simulink model "gm_uz_pmsm_model_9ph_vnl"  (R2021b)
settings: Solver=FixedStepAuto  StartTime=0.0  StopTime=0.8  RelTol=1e-3
PreLoadFcn:
  | uz_pmsm_model_9ph_init_parameter
undefined symbols (not defined in the file or in its folder): a, b, c, friction_coefficient, inertia, k_i_d, k_i_q, k_p_d, k_p_q, Kpd, L_d, L_o1, L_o2, L_q, L_x1, L_x2, L_y1, L_y2, L_zero, polepair, psi_pm, R_1, static_friction_torque, Tnd, ts
libraries: hdlmdlgenlib x191, hdlsllib x90, dspsigops x19, simulink x17, slpidlib x2, spsAlphaBetaZerotodq0Lib x1, pid_lib x1, spsdq0toAlphaBetaZeroLib x1
(part 5 of 7)

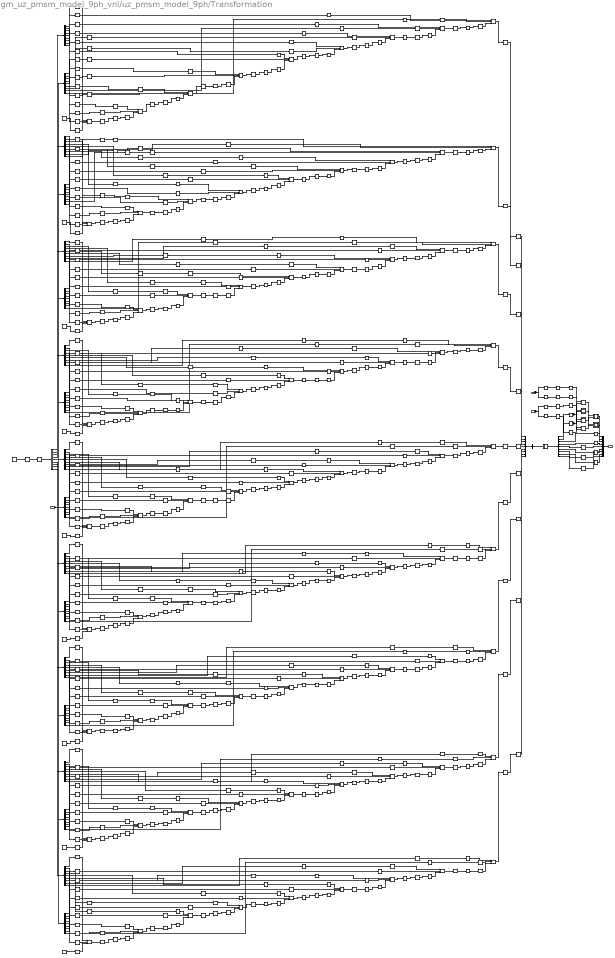
== system gm_uz_pmsm_model_9ph_vnl/uz_pmsm_model_9ph/Transformation ==
  in : Inport  OutDataTypeStr=fixdt(1, 25, 12)  PortDimensions=[9]  SampleTime=1e-08
  sin_theta_el : Inport  Port=2  OutDataTypeStr=single  SampleTime=1e-08
  cos_theta_el : Inport  Port=3  OutDataTypeStr=single  SampleTime=1e-08
  Add : Subsystem
      mask Display: disp('NFP\nadd');
  Add1 : Subsystem
      mask Display: disp('NFP\nadd');
  Constant1 : Constant  Value=[0.22222137451171875;0;0.22222137451171875;0;0.22222137451171875;0;0.22222137451171875;0;0.111110687255859375;-0.111110687255859375;0.1924495697021484375;0.22222137451171875;0;-0.111110687255859375;-0.1924495697021484375;-0.111110687255859375;0.1924495697021484375;0.111110687255859375;-0.111110687255859375;-0.1924495697021484375;0.22222137451171875;0;-0.111110687255859375;0.1924495697021484375;-0.111110687255859375;-0.1924495697021484375;0.111110687255859375;0.208820343017578125;0.0760040283203125;0.111110687255859375;0.1924495697021484375;-0.0385875701904296875;0.218845367431640625;-0.1702327728271484375;0.142841339111328125;-0.111110687255859375;-0.1702327728271484375;0.142841339111328125;0.111110687255859375;0.1924495697021484375;0.208820343017578125;-0.0760040283203125;-0.0385875701904296875;-0.218845367431640625;-0.111110687255859375;-0.0385875701904296875;-0.218845367431640625;0.111110687255859375;0.1924495697021484375;-0.1702327728271484375;-0.142841339111328125;0.208820343017578125;0.0760040283203125;-0.111110687255859375;0.1702327728271484375;0.142841339111328125;-0.111110687255859375;0.1924495697021484375;-0.208820343017578125;-0.0760040283203125;0.0385875701904296875;-0.218845367431640625;0.111110687255859375;-0.208820343017578125;0.0760040283203125;-0.111110687255859375;0.1924495697021484375;0.0385875701904296875;0.218845367431640625;0.1702327728271484375;0.142841339111328125;0.111110687255859375;0.0385875701904296875;-0.218845367431640625;-0.111110687255859375;0.1924495697021484375;0.1702327728271484375;-0.142841339111328125;-0.208820343017578125;0.0760040283203125;0.111110687255859375]  OutDataTypeStr=fixdt(1, 18, 19)  SampleTime=1e-08
  Data Type Conversion39 : Subsystem
      mask Display: disp('NFP\nconv');
  Data Type Conversion39_out1_0_wire : hdlmdlgenlib/Buffer
      settings: SourceProductBaseCode=SL
  Data Type Conversion39_out1_1_wire : hdlmdlgenlib/Buffer
      settings: SourceProductBaseCode=SL
  Divide : Subsystem
      mask Display: disp('NFP\nmul');
  Divide1 : Subsystem
      mask Display: disp('NFP\nmul');
  Divide2 : Subsystem
      mask Display: disp('NFP\nmul');
  Divide3 : Subsystem
      mask Display: disp('NFP\nmul');
  From{1..2,17..18} (4 alike) : hdlmdlgenlib/Buffer
      settings: SourceProductBaseCode=SL
  HwModeRegister{,1..242} (243 alike) : Delay  DelayLength=double(1)  InitialCondition=0  SampleTime=1e-08
  PipelineRegister{,1..80} (81 alike) : Delay  DelayLength=double(2)  InitialCondition=0  SampleTime=1e-08
  _adder_MultiplyAdd{,1..80} (81 alike) : hdlsllib/HDL Operations/Multiply-Add  Function=c+(a.*b)  datatype=fixdt(1, 44, 31)  DoSatur=off  FMA=off
      settings: SourceProductBaseCode=SL
  _adder_MultiplyAdd_out_dtc{,1..80} (81 alike) : DataTypeConversion  OutDataTypeStr=fixdt(1, 43, 31)  SampleTime=1e-08
  _bias{,1..8} (9 alike) : Constant  Value=double(0)  OutDataTypeStr=fixdt(1, 43, 31)  SampleTime=1e-08
  delayMatch{,1,14..15,28..29,42..43,56..57,70..71,84..85,98..99,112..113} (18 alike) : Delay  DelayLength=double(3)  InitialCondition=0  SampleTime=1e-08
  delayMatch{10..11,24..25,38..39,52..53,66..67,80..81,94..95,108..109,122..123} (18 alike) : Delay  DelayLength=double(18)  InitialCondition=0  SampleTime=1e-08
  delayMatch{2..3,16..17,30..31,44..45,58..59,72..73,86..87,100..101,114..115,148..151} (22 alike) : Delay  DelayLength=double(6)  InitialCondition=0  SampleTime=1e-08
  delayMatch{4..5,18..19,32..33,46..47,60..61,74..75,88..89,102..103,116..117} (18 alike) : Delay  DelayLength=double(9)  InitialCondition=0  SampleTime=1e-08
  delayMatch{6..7,20..21,34..35,48..49,62..63,76..77,90..91,104..105,118..119,152..158} (25 alike) : Delay  DelayLength=double(12)  InitialCondition=0  SampleTime=1e-08
  delayMatch{8..9,22..23,36..37,50..51,64..65,78..79,92..93,106..107,120..121} (18 alike) : Delay  DelayLength=double(15)  InitialCondition=0  SampleTime=1e-08
  delayMatch{12..13,26..27,40..41,54..55,68..69,82..83,96..97,110..111,124..125} (18 alike) : Delay  DelayLength=double(21)  InitialCondition=0  SampleTime=1e-08
  delayMatch{126..143} (18 alike) : Delay  DelayLength=double(24)  InitialCondition=0  SampleTime=1e-08
  delayMatch{144..147} (4 alike) : Delay  DelayLength=double(27)  InitialCondition=0  SampleTime=1e-08
  mux : Mux  Inputs=9
  t{,6..23} (19 alike) : Demux  Outputs=9
  t1 : Reshape  OutputDimensionality=Customize  OutputDimensions=[9,9]
  t2 : Math  Operator=transpose  SaturateOnIntegerOverflow=on
  t3 : Subsystem
  t4 : Mux  Inputs=9
  t5 : Concatenate  NumInputs=1  Mode=Multidimensional array  ConcatenateDimension=2
  out : Outport  SampleTime=1e-08
  wires:
  HwModeRegister242/1 -> _adder_MultiplyAdd80/3
  HwModeRegister241/1 -> _adder_MultiplyAdd80/2
  HwModeRegister240/1 -> _adder_MultiplyAdd80/1
  _adder_MultiplyAdd80/1 -> PipelineRegister80/1
  HwModeRegister239/1 -> _adder_MultiplyAdd79/3
  HwModeRegister238/1 -> _adder_MultiplyAdd79/2
  HwModeRegister237/1 -> _adder_MultiplyAdd79/1
  _adder_MultiplyAdd79/1 -> PipelineRegister79/1
  HwModeRegister236/1 -> _adder_MultiplyAdd78/3
  HwModeRegister235/1 -> _adder_MultiplyAdd78/2
  HwModeRegister234/1 -> _adder_MultiplyAdd78/1
  _adder_MultiplyAdd78/1 -> PipelineRegister78/1
  HwModeRegister233/1 -> _adder_MultiplyAdd77/3
  HwModeRegister232/1 -> _adder_MultiplyAdd77/2
  HwModeRegister231/1 -> _adder_MultiplyAdd77/1
  _adder_MultiplyAdd77/1 -> PipelineRegister77/1
  HwModeRegister230/1 -> _adder_MultiplyAdd76/3
  HwModeRegister229/1 -> _adder_MultiplyAdd76/2
  HwModeRegister228/1 -> _adder_MultiplyAdd76/1
  _adder_MultiplyAdd76/1 -> PipelineRegister76/1
  HwModeRegister227/1 -> _adder_MultiplyAdd75/3
  HwModeRegister226/1 -> _adder_MultiplyAdd75/2
  HwModeRegister225/1 -> _adder_MultiplyAdd75/1
  _adder_MultiplyAdd75/1 -> PipelineRegister75/1
  HwModeRegister224/1 -> _adder_MultiplyAdd74/3
  HwModeRegister223/1 -> _adder_MultiplyAdd74/2
  HwModeRegister222/1 -> _adder_MultiplyAdd74/1
  _adder_MultiplyAdd74/1 -> PipelineRegister74/1
  HwModeRegister221/1 -> _adder_MultiplyAdd73/3
  HwModeRegister220/1 -> _adder_MultiplyAdd73/2
  HwModeRegister219/1 -> _adder_MultiplyAdd73/1
  _adder_MultiplyAdd73/1 -> PipelineRegister73/1
  HwModeRegister218/1 -> _adder_MultiplyAdd72/3
  HwModeRegister217/1 -> _adder_MultiplyAdd72/2
  HwModeRegister216/1 -> _adder_MultiplyAdd72/1
  _adder_MultiplyAdd72/1 -> PipelineRegister72/1
  HwModeRegister215/1 -> _adder_MultiplyAdd71/3
  HwModeRegister214/1 -> _adder_MultiplyAdd71/2
  HwModeRegister213/1 -> _adder_MultiplyAdd71/1
  _adder_MultiplyAdd71/1 -> PipelineRegister71/1
  HwModeRegister212/1 -> _adder_MultiplyAdd70/3
  HwModeRegister211/1 -> _adder_MultiplyAdd70/2
  HwModeRegister210/1 -> _adder_MultiplyAdd70/1
  _adder_MultiplyAdd70/1 -> PipelineRegister70/1
  HwModeRegister209/1 -> _adder_MultiplyAdd69/3
  HwModeRegister208/1 -> _adder_MultiplyAdd69/2
  HwModeRegister207/1 -> _adder_MultiplyAdd69/1
  _adder_MultiplyAdd69/1 -> PipelineRegister69/1
  HwModeRegister206/1 -> _adder_MultiplyAdd68/3
  HwModeRegister205/1 -> _adder_MultiplyAdd68/2
  HwModeRegister204/1 -> _adder_MultiplyAdd68/1
  _adder_MultiplyAdd68/1 -> PipelineRegister68/1
  HwModeRegister203/1 -> _adder_MultiplyAdd67/3
  HwModeRegister202/1 -> _adder_MultiplyAdd67/2
  HwModeRegister201/1 -> _adder_MultiplyAdd67/1
  _adder_MultiplyAdd67/1 -> PipelineRegister67/1
  HwModeRegister200/1 -> _adder_MultiplyAdd66/3
  HwModeRegister199/1 -> _adder_MultiplyAdd66/2
  HwModeRegister198/1 -> _adder_MultiplyAdd66/1
  _adder_MultiplyAdd66/1 -> PipelineRegister66/1
  HwModeRegister197/1 -> _adder_MultiplyAdd65/3
  HwModeRegister196/1 -> _adder_MultiplyAdd65/2
  HwModeRegister195/1 -> _adder_MultiplyAdd65/1
  _adder_MultiplyAdd65/1 -> PipelineRegister65/1
  HwModeRegister194/1 -> _adder_MultiplyAdd64/3
  HwModeRegister193/1 -> _adder_MultiplyAdd64/2
  HwModeRegister192/1 -> _adder_MultiplyAdd64/1
  _adder_MultiplyAdd64/1 -> PipelineRegister64/1
  HwModeRegister191/1 -> _adder_MultiplyAdd63/3
  HwModeRegister190/1 -> _adder_MultiplyAdd63/2
  HwModeRegister189/1 -> _adder_MultiplyAdd63/1
  _adder_MultiplyAdd63/1 -> PipelineRegister63/1
  HwModeRegister188/1 -> _adder_MultiplyAdd62/3
  HwModeRegister187/1 -> _adder_MultiplyAdd62/2
  HwModeRegister186/1 -> _adder_MultiplyAdd62/1
  _adder_MultiplyAdd62/1 -> PipelineRegister62/1
  HwModeRegister185/1 -> _adder_MultiplyAdd61/3
  HwModeRegister184/1 -> _adder_MultiplyAdd61/2
  HwModeRegister183/1 -> _adder_MultiplyAdd61/1
  _adder_MultiplyAdd61/1 -> PipelineRegister61/1
  HwModeRegister182/1 -> _adder_MultiplyAdd60/3
  HwModeRegister181/1 -> _adder_MultiplyAdd60/2
  HwModeRegister180/1 -> _adder_MultiplyAdd60/1
  _adder_MultiplyAdd60/1 -> PipelineRegister60/1
  HwModeRegister179/1 -> _adder_MultiplyAdd59/3
  HwModeRegister178/1 -> _adder_MultiplyAdd59/2
  HwModeRegister177/1 -> _adder_MultiplyAdd59/1
  _adder_MultiplyAdd59/1 -> PipelineRegister59/1
  HwModeRegister176/1 -> _adder_MultiplyAdd58/3
  HwModeRegister175/1 -> _adder_MultiplyAdd58/2
  HwModeRegister174/1 -> _adder_MultiplyAdd58/1
  _adder_MultiplyAdd58/1 -> PipelineRegister58/1
  HwModeRegister173/1 -> _adder_MultiplyAdd57/3
  HwModeRegister172/1 -> _adder_MultiplyAdd57/2
  HwModeRegister171/1 -> _adder_MultiplyAdd57/1
  _adder_MultiplyAdd57/1 -> PipelineRegister57/1
  HwModeRegister170/1 -> _adder_MultiplyAdd56/3
  HwModeRegister169/1 -> _adder_MultiplyAdd56/2
  HwModeRegister168/1 -> _adder_MultiplyAdd56/1
  _adder_MultiplyAdd56/1 -> PipelineRegister56/1
  HwModeRegister167/1 -> _adder_MultiplyAdd55/3
  HwModeRegister166/1 -> _adder_MultiplyAdd55/2
  HwModeRegister165/1 -> _adder_MultiplyAdd55/1
  _adder_MultiplyAdd55/1 -> PipelineRegister55/1
  HwModeRegister164/1 -> _adder_MultiplyAdd54/3
  HwModeRegister163/1 -> _adder_MultiplyAdd54/2
  HwModeRegister162/1 -> _adder_MultiplyAdd54/1
  _adder_MultiplyAdd54/1 -> PipelineRegister54/1
  HwModeRegister161/1 -> _adder_MultiplyAdd53/3
  HwModeRegister160/1 -> _adder_MultiplyAdd53/2
  HwModeRegister159/1 -> _adder_MultiplyAdd53/1
  _adder_MultiplyAdd53/1 -> PipelineRegister53/1
  HwModeRegister158/1 -> _adder_MultiplyAdd52/3
  HwModeRegister157/1 -> _adder_MultiplyAdd52/2
  HwModeRegister156/1 -> _adder_MultiplyAdd52/1
  _adder_MultiplyAdd52/1 -> PipelineRegister52/1
  HwModeRegister155/1 -> _adder_MultiplyAdd51/3
  HwModeRegister154/1 -> _adder_MultiplyAdd51/2
  HwModeRegister153/1 -> _adder_MultiplyAdd51/1
  _adder_MultiplyAdd51/1 -> PipelineRegister51/1
  HwModeRegister152/1 -> _adder_MultiplyAdd50/3
  HwModeRegister151/1 -> _adder_MultiplyAdd50/2
  HwModeRegister150/1 -> _adder_MultiplyAdd50/1
  _adder_MultiplyAdd50/1 -> PipelineRegister50/1
  HwModeRegister149/1 -> _adder_MultiplyAdd49/3
  HwModeRegister148/1 -> _adder_MultiplyAdd49/2
  HwModeRegister147/1 -> _adder_MultiplyAdd49/1
  _adder_MultiplyAdd49/1 -> PipelineRegister49/1
  HwModeRegister146/1 -> _adder_MultiplyAdd48/3
  HwModeRegister145/1 -> _adder_MultiplyAdd48/2
  HwModeRegister144/1 -> _adder_MultiplyAdd48/1
  _adder_MultiplyAdd48/1 -> PipelineRegister48/1
  HwModeRegister143/1 -> _adder_MultiplyAdd47/3
  HwModeRegister142/1 -> _adder_MultiplyAdd47/2
  HwModeRegister141/1 -> _adder_MultiplyAdd47/1
  _adder_MultiplyAdd47/1 -> PipelineRegister47/1
  HwModeRegister140/1 -> _adder_MultiplyAdd46/3
  HwModeRegister139/1 -> _adder_MultiplyAdd46/2
  HwModeRegister138/1 -> _adder_MultiplyAdd46/1
  _adder_MultiplyAdd46/1 -> PipelineRegister46/1
  HwModeRegister137/1 -> _adder_MultiplyAdd45/3
  HwModeRegister136/1 -> _adder_MultiplyAdd45/2
  HwModeRegister135/1 -> _adder_MultiplyAdd45/1
  _adder_MultiplyAdd45/1 -> PipelineRegister45/1
  HwModeRegister134/1 -> _adder_MultiplyAdd44/3
  HwModeRegister133/1 -> _adder_MultiplyAdd44/2
  HwModeRegister132/1 -> _adder_MultiplyAdd44/1
  _adder_MultiplyAdd44/1 -> PipelineRegister44/1
  HwModeRegister131/1 -> _adder_MultiplyAdd43/3
  HwModeRegister130/1 -> _adder_MultiplyAdd43/2
  HwModeRegister129/1 -> _adder_MultiplyAdd43/1
  _adder_MultiplyAdd43/1 -> PipelineRegister43/1
  HwModeRegister128/1 -> _adder_MultiplyAdd42/3
  HwModeRegister127/1 -> _adder_MultiplyAdd42/2
  HwModeRegister126/1 -> _adder_MultiplyAdd42/1
  _adder_MultiplyAdd42/1 -> PipelineRegister42/1
  HwModeRegister125/1 -> _adder_MultiplyAdd41/3
  HwModeRegister124/1 -> _adder_MultiplyAdd41/2
  HwModeRegister123/1 -> _adder_MultiplyAdd41/1
  _adder_MultiplyAdd41/1 -> PipelineRegister41/1
  HwModeRegister122/1 -> _adder_MultiplyAdd40/3
  HwModeRegister121/1 -> _adder_MultiplyAdd40/2
  HwModeRegister120/1 -> _adder_MultiplyAdd40/1
  _adder_MultiplyAdd40/1 -> PipelineRegister40/1
  HwModeRegister119/1 -> _adder_MultiplyAdd39/3
  HwModeRegister118/1 -> _adder_MultiplyAdd39/2
  HwModeRegister117/1 -> _adder_MultiplyAdd39/1
  _adder_MultiplyAdd39/1 -> PipelineRegister39/1
  HwModeRegister116/1 -> _adder_MultiplyAdd38/3
  HwModeRegister115/1 -> _adder_MultiplyAdd38/2
  HwModeRegister114/1 -> _adder_MultiplyAdd38/1
  _adder_MultiplyAdd38/1 -> PipelineRegister38/1
  HwModeRegister113/1 -> _adder_MultiplyAdd37/3
  HwModeRegister112/1 -> _adder_MultiplyAdd37/2
  HwModeRegister111/1 -> _adder_MultiplyAdd37/1
  _adder_MultiplyAdd37/1 -> PipelineRegister37/1
  HwModeRegister110/1 -> _adder_MultiplyAdd36/3
  HwModeRegister109/1 -> _adder_MultiplyAdd36/2
  HwModeRegister108/1 -> _adder_MultiplyAdd36/1
  _adder_MultiplyAdd36/1 -> PipelineRegister36/1
  HwModeRegister107/1 -> _adder_MultiplyAdd35/3
  HwModeRegister106/1 -> _adder_MultiplyAdd35/2
  HwModeRegister105/1 -> _adder_MultiplyAdd35/1
  _adder_MultiplyAdd35/1 -> PipelineRegister35/1
  HwModeRegister104/1 -> _adder_MultiplyAdd34/3
  HwModeRegister103/1 -> _adder_MultiplyAdd34/2
  HwModeRegister102/1 -> _adder_MultiplyAdd34/1
  _adder_MultiplyAdd34/1 -> PipelineRegister34/1
  HwModeRegister101/1 -> _adder_MultiplyAdd33/3
  HwModeRegister100/1 -> _adder_MultiplyAdd33/2
  HwModeRegister99/1 -> _adder_MultiplyAdd33/1
  _adder_MultiplyAdd33/1 -> PipelineRegister33/1
  HwModeRegister98/1 -> _adder_MultiplyAdd32/3
  HwModeRegister97/1 -> _adder_MultiplyAdd32/2
  HwModeRegister96/1 -> _adder_MultiplyAdd32/1
  _adder_MultiplyAdd32/1 -> PipelineRegister32/1
  HwModeRegister95/1 -> _adder_MultiplyAdd31/3
  HwModeRegister94/1 -> _adder_MultiplyAdd31/2
  HwModeRegister93/1 -> _adder_MultiplyAdd31/1
  _adder_MultiplyAdd31/1 -> PipelineRegister31/1
  HwModeRegister92/1 -> _adder_MultiplyAdd30/3
  HwModeRegister91/1 -> _adder_MultiplyAdd30/2
  HwModeRegister90/1 -> _adder_MultiplyAdd30/1
  _adder_MultiplyAdd30/1 -> PipelineRegister30/1
  HwModeRegister89/1 -> _adder_MultiplyAdd29/3
  HwModeRegister88/1 -> _adder_MultiplyAdd29/2
  HwModeRegister87/1 -> _adder_MultiplyAdd29/1
  _adder_MultiplyAdd29/1 -> PipelineRegister29/1
  HwModeRegister86/1 -> _adder_MultiplyAdd28/3
  HwModeRegister85/1 -> _adder_MultiplyAdd28/2
  HwModeRegister84/1 -> _adder_MultiplyAdd28/1
  _adder_MultiplyAdd28/1 -> PipelineRegister28/1
  HwModeRegister83/1 -> _adder_MultiplyAdd27/3
  HwModeRegister82/1 -> _adder_MultiplyAdd27/2
  HwModeRegister81/1 -> _adder_MultiplyAdd27/1
  _adder_MultiplyAdd27/1 -> PipelineRegister27/1
  HwModeRegister80/1 -> _adder_MultiplyAdd26/3
  HwModeRegister79/1 -> _adder_MultiplyAdd26/2
  HwModeRegister78/1 -> _adder_MultiplyAdd26/1
  _adder_MultiplyAdd26/1 -> PipelineRegister26/1
  HwModeRegister77/1 -> _adder_MultiplyAdd25/3
  HwModeRegister76/1 -> _adder_MultiplyAdd25/2
  HwModeRegister75/1 -> _adder_MultiplyAdd25/1
  _adder_MultiplyAdd25/1 -> PipelineRegister25/1
  HwModeRegister74/1 -> _adder_MultiplyAdd24/3
  HwModeRegister73/1 -> _adder_MultiplyAdd24/2
  HwModeRegister72/1 -> _adder_MultiplyAdd24/1
  _adder_MultiplyAdd24/1 -> PipelineRegister24/1
  HwModeRegister71/1 -> _adder_MultiplyAdd23/3
  HwModeRegister70/1 -> _adder_MultiplyAdd23/2
  HwModeRegister69/1 -> _adder_MultiplyAdd23/1
  _adder_MultiplyAdd23/1 -> PipelineRegister23/1
  HwModeRegister68/1 -> _adder_MultiplyAdd22/3
  HwModeRegister67/1 -> _adder_MultiplyAdd22/2
  HwModeRegister66/1 -> _adder_MultiplyAdd22/1
  _adder_MultiplyAdd22/1 -> PipelineRegister22/1
  HwModeRegister65/1 -> _adder_MultiplyAdd21/3
  HwModeRegister64/1 -> _adder_MultiplyAdd21/2
  HwModeRegister63/1 -> _adder_MultiplyAdd21/1
  _adder_MultiplyAdd21/1 -> PipelineRegister21/1
  HwModeRegister62/1 -> _adder_MultiplyAdd20/3
  HwModeRegister61/1 -> _adder_MultiplyAdd20/2
  HwModeRegister60/1 -> _adder_MultiplyAdd20/1
  _adder_MultiplyAdd20/1 -> PipelineRegister20/1
  HwModeRegister59/1 -> _adder_MultiplyAdd19/3
  HwModeRegister58/1 -> _adder_MultiplyAdd19/2
  HwModeRegister57/1 -> _adder_MultiplyAdd19/1
  _adder_MultiplyAdd19/1 -> PipelineRegister19/1
  HwModeRegister56/1 -> _adder_MultiplyAdd18/3
  HwModeRegister55/1 -> _adder_MultiplyAdd18/2
  HwModeRegister54/1 -> _adder_MultiplyAdd18/1
  _adder_MultiplyAdd18/1 -> PipelineRegister18/1
  HwModeRegister53/1 -> _adder_MultiplyAdd17/3
  HwModeRegister52/1 -> _adder_MultiplyAdd17/2
  HwModeRegister51/1 -> _adder_MultiplyAdd17/1
  _adder_MultiplyAdd17/1 -> PipelineRegister17/1
  HwModeRegister50/1 -> _adder_MultiplyAdd16/3
  HwModeRegister49/1 -> _adder_MultiplyAdd16/2
  HwModeRegister48/1 -> _adder_MultiplyAdd16/1
  _adder_MultiplyAdd16/1 -> PipelineRegister16/1
  HwModeRegister47/1 -> _adder_MultiplyAdd15/3
  HwModeRegister46/1 -> _adder_MultiplyAdd15/2
  HwModeRegister45/1 -> _adder_MultiplyAdd15/1
  _adder_MultiplyAdd15/1 -> PipelineRegister15/1
  HwModeRegister44/1 -> _adder_MultiplyAdd14/3
  HwModeRegister43/1 -> _adder_MultiplyAdd14/2
  HwModeRegister42/1 -> _adder_MultiplyAdd14/1
  _adder_MultiplyAdd14/1 -> PipelineRegister14/1
  HwModeRegister41/1 -> _adder_MultiplyAdd13/3
  HwModeRegister40/1 -> _adder_MultiplyAdd13/2
  HwModeRegister39/1 -> _adder_MultiplyAdd13/1
  _adder_MultiplyAdd13/1 -> PipelineRegister13/1
  HwModeRegister38/1 -> _adder_MultiplyAdd12/3
  HwModeRegister37/1 -> _adder_MultiplyAdd12/2
  HwModeRegister36/1 -> _adder_MultiplyAdd12/1
  _adder_MultiplyAdd12/1 -> PipelineRegister12/1
  HwModeRegister35/1 -> _adder_MultiplyAdd11/3
  HwModeRegister34/1 -> _adder_MultiplyAdd11/2
  HwModeRegister33/1 -> _adder_MultiplyAdd11/1
  _adder_MultiplyAdd11/1 -> PipelineRegister11/1
  HwModeRegister32/1 -> _adder_MultiplyAdd10/3
  HwModeRegister31/1 -> _adder_MultiplyAdd10/2
  HwModeRegister30/1 -> _adder_MultiplyAdd10/1
  _adder_MultiplyAdd10/1 -> PipelineRegister10/1
  HwModeRegister29/1 -> _adder_MultiplyAdd9/3
  HwModeRegister28/1 -> _adder_MultiplyAdd9/2
  HwModeRegister27/1 -> _adder_MultiplyAdd9/1
  _adder_MultiplyAdd9/1 -> PipelineRegister9/1
  HwModeRegister26/1 -> _adder_MultiplyAdd8/3
  HwModeRegister25/1 -> _adder_MultiplyAdd8/2
  HwModeRegister24/1 -> _adder_MultiplyAdd8/1
  _adder_MultiplyAdd8/1 -> PipelineRegister8/1
  HwModeRegister23/1 -> _adder_MultiplyAdd7/3
  HwModeRegister22/1 -> _adder_MultiplyAdd7/2
  HwModeRegister21/1 -> _adder_MultiplyAdd7/1
  _adder_MultiplyAdd7/1 -> PipelineRegister7/1
  HwModeRegister20/1 -> _adder_MultiplyAdd6/3
  HwModeRegister19/1 -> _adder_MultiplyAdd6/2
  HwModeRegister18/1 -> _adder_MultiplyAdd6/1
  _adder_MultiplyAdd6/1 -> PipelineRegister6/1
  HwModeRegister17/1 -> _adder_MultiplyAdd5/3
  HwModeRegister16/1 -> _adder_MultiplyAdd5/2
  HwModeRegister15/1 -> _adder_MultiplyAdd5/1
  _adder_MultiplyAdd5/1 -> PipelineRegister5/1
  HwModeRegister14/1 -> _adder_MultiplyAdd4/3
  HwModeRegister13/1 -> _adder_MultiplyAdd4/2
  HwModeRegister12/1 -> _adder_MultiplyAdd4/1
  _adder_MultiplyAdd4/1 -> PipelineRegister4/1
  HwModeRegister11/1 -> _adder_MultiplyAdd3/3
  HwModeRegister10/1 -> _adder_MultiplyAdd3/2
  HwModeRegister9/1 -> _adder_MultiplyAdd3/1
  _adder_MultiplyAdd3/1 -> PipelineRegister3/1
  HwModeRegister8/1 -> _adder_MultiplyAdd2/3
  HwModeRegister7/1 -> _adder_MultiplyAdd2/2
  HwModeRegister6/1 -> _adder_MultiplyAdd2/1
  _adder_MultiplyAdd2/1 -> PipelineRegister2/1
  HwModeRegister5/1 -> _adder_MultiplyAdd1/3
  HwModeRegister4/1 -> _adder_MultiplyAdd1/2
  HwModeRegister3/1 -> _adder_MultiplyAdd1/1
  _adder_MultiplyAdd1/1 -> PipelineRegister1/1
  HwModeRegister2/1 -> _adder_MultiplyAdd/3
  HwModeRegister1/1 -> _adder_MultiplyAdd/2
  HwModeRegister/1 -> _adder_MultiplyAdd/1
  _adder_MultiplyAdd/1 -> PipelineRegister/1
  cos_theta_el/1 -> From17/1, From2/1
  sin_theta_el/1 -> From1/1, From18/1
  in/1 -> t7/1, t9/1, t11/1, t13/1, t15/1, t17/1, t19/1, t21/1, t23/1
  delayMatch147/1 -> delayMatch151/1
  delayMatch145/1 -> delayMatch150/1
  delayMatch146/1 -> delayMatch149/1
  delayMatch144/1 -> delayMatch148/1
  Divide3/1(Out1) -> Add1/1(In1)
  Divide2/1(Out1) -> Add1/2(In2)
  Divide1/1(Out1) -> Add/2(In2)
  Divide/1(Out1) -> Add/1(In1)
  Data Type Conversion39/1(Out1) -> t/1
  Add1/1(Out1) -> mux/2
  Add/1(Out1) -> mux/1
  From1/1 -> delayMatch147/1
  From18/1 -> delayMatch146/1
  From2/1 -> delayMatch145/1
  From17/1 -> delayMatch144/1
  t23/9 -> delayMatch143/1
  t22/9 -> delayMatch142/1
  t21/9 -> delayMatch141/1
  t20/9 -> delayMatch140/1
  t19/9 -> delayMatch139/1
  t18/9 -> delayMatch138/1
  t17/9 -> delayMatch137/1
  t16/9 -> delayMatch136/1
  t15/9 -> delayMatch135/1
  t14/9 -> delayMatch134/1
  t13/9 -> delayMatch133/1
  t12/9 -> delayMatch132/1
  t11/9 -> delayMatch131/1
  t10/9 -> delayMatch130/1
  t9/9 -> delayMatch129/1
  t8/9 -> delayMatch128/1
  t7/9 -> delayMatch127/1
  t6/9 -> delayMatch126/1
  t23/8 -> delayMatch125/1
  t22/8 -> delayMatch124/1
  t23/7 -> delayMatch123/1
  t22/7 -> delayMatch122/1
  t23/6 -> delayMatch121/1
  t22/6 -> delayMatch120/1
  t23/5 -> delayMatch119/1
  t22/5 -> delayMatch118/1
  t23/4 -> delayMatch117/1
  t22/4 -> delayMatch116/1
  t23/3 -> delayMatch115/1
  t22/3 -> delayMatch114/1
  t23/2 -> delayMatch113/1
  t22/2 -> delayMatch112/1
  t21/8 -> delayMatch111/1
  t20/8 -> delayMatch110/1
  t21/7 -> delayMatch109/1
  t20/7 -> delayMatch108/1
  t21/6 -> delayMatch107/1
  t20/6 -> delayMatch106/1
  t21/5 -> delayMatch105/1
  t20/5 -> delayMatch104/1
  t21/4 -> delayMatch103/1
  t20/4 -> delayMatch102/1
  t21/3 -> delayMatch101/1
  t20/3 -> delayMatch100/1
  t21/2 -> delayMatch99/1
  t20/2 -> delayMatch98/1
  t19/8 -> delayMatch97/1
  t18/8 -> delayMatch96/1
  t19/7 -> delayMatch95/1
  t18/7 -> delayMatch94/1
  t19/6 -> delayMatch93/1
  t18/6 -> delayMatch92/1
  t19/5 -> delayMatch91/1
  t18/5 -> delayMatch90/1
  t19/4 -> delayMatch89/1
  t18/4 -> delayMatch88/1
  t19/3 -> delayMatch87/1
  t18/3 -> delayMatch86/1
  t19/2 -> delayMatch85/1
  t18/2 -> delayMatch84/1
  t17/8 -> delayMatch83/1
  t16/8 -> delayMatch82/1
  t17/7 -> delayMatch81/1
  t16/7 -> delayMatch80/1
  t17/6 -> delayMatch79/1
  t16/6 -> delayMatch78/1
  t17/5 -> delayMatch77/1
  t16/5 -> delayMatch76/1
  t17/4 -> delayMatch75/1
  t16/4 -> delayMatch74/1
  t17/3 -> delayMatch73/1
  t16/3 -> delayMatch72/1
  t17/2 -> delayMatch71/1
  t16/2 -> delayMatch70/1
  t15/8 -> delayMatch69/1
  t14/8 -> delayMatch68/1
  t15/7 -> delayMatch67/1
  t14/7 -> delayMatch66/1
  t15/6 -> delayMatch65/1
  t14/6 -> delayMatch64/1
  t15/5 -> delayMatch63/1
  t14/5 -> delayMatch62/1
  t15/4 -> delayMatch61/1
  t14/4 -> delayMatch60/1
  t15/3 -> delayMatch59/1
  t14/3 -> delayMatch58/1
  t15/2 -> delayMatch57/1
  t14/2 -> delayMatch56/1
  t13/8 -> delayMatch55/1
  t12/8 -> delayMatch54/1
  t13/7 -> delayMatch53/1
  t12/7 -> delayMatch52/1
  t13/6 -> delayMatch51/1
  t12/6 -> delayMatch50/1
  t13/5 -> delayMatch49/1
  t12/5 -> delayMatch48/1
  t13/4 -> delayMatch47/1
  t12/4 -> delayMatch46/1
  t13/3 -> delayMatch45/1
  t12/3 -> delayMatch44/1
  t13/2 -> delayMatch43/1
  t12/2 -> delayMatch42/1
  t11/8 -> delayMatch41/1
  t10/8 -> delayMatch40/1
  t11/7 -> delayMatch39/1
  t10/7 -> delayMatch38/1
  t11/6 -> delayMatch37/1
  t10/6 -> delayMatch36/1
  t11/5 -> delayMatch35/1
  t10/5 -> delayMatch34/1
  t11/4 -> delayMatch33/1
  t10/4 -> delayMatch32/1
  t11/3 -> delayMatch31/1
  t10/3 -> delayMatch30/1
  t11/2 -> delayMatch29/1
  t10/2 -> delayMatch28/1
  t9/8 -> delayMatch27/1
  t8/8 -> delayMatch26/1
  t9/7 -> delayMatch25/1
  t8/7 -> delayMatch24/1
  t9/6 -> delayMatch23/1
  t8/6 -> delayMatch22/1
  t9/5 -> delayMatch21/1
  t8/5 -> delayMatch20/1
  t9/4 -> delayMatch19/1
  t8/4 -> delayMatch18/1
  t9/3 -> delayMatch17/1
  t8/3 -> delayMatch16/1
  t9/2 -> delayMatch15/1
  t8/2 -> delayMatch14/1
  t7/8 -> delayMatch13/1
  t6/8 -> delayMatch12/1
  t7/7 -> delayMatch11/1
  t6/7 -> delayMatch10/1
  t7/6 -> delayMatch9/1
  t6/6 -> delayMatch8/1
  t7/5 -> delayMatch7/1
  t6/5 -> delayMatch6/1
  t7/4 -> delayMatch5/1
  t6/4 -> delayMatch4/1
  t7/3 -> delayMatch3/1
  t6/3 -> delayMatch2/1
  t7/2 -> delayMatch1/1
  t6/2 -> delayMatch/1
  PipelineRegister80/1 -> _adder_MultiplyAdd_out_dtc80/1
  PipelineRegister79/1 -> _adder_MultiplyAdd_out_dtc79/1
  PipelineRegister78/1 -> _adder_MultiplyAdd_out_dtc78/1
  PipelineRegister77/1 -> _adder_MultiplyAdd_out_dtc77/1
  PipelineRegister76/1 -> _adder_MultiplyAdd_out_dtc76/1
  PipelineRegister75/1 -> _adder_MultiplyAdd_out_dtc75/1
  PipelineRegister74/1 -> _adder_MultiplyAdd_out_dtc74/1
  PipelineRegister73/1 -> _adder_MultiplyAdd_out_dtc73/1
  PipelineRegister72/1 -> _adder_MultiplyAdd_out_dtc72/1
  PipelineRegister71/1 -> _adder_MultiplyAdd_out_dtc71/1
  PipelineRegister70/1 -> _adder_MultiplyAdd_out_dtc70/1
  PipelineRegister69/1 -> _adder_MultiplyAdd_out_dtc69/1
  PipelineRegister68/1 -> _adder_MultiplyAdd_out_dtc68/1
  PipelineRegister67/1 -> _adder_MultiplyAdd_out_dtc67/1
  PipelineRegister66/1 -> _adder_MultiplyAdd_out_dtc66/1
  PipelineRegister65/1 -> _adder_MultiplyAdd_out_dtc65/1
  PipelineRegister64/1 -> _adder_MultiplyAdd_out_dtc64/1
  PipelineRegister63/1 -> _adder_MultiplyAdd_out_dtc63/1
  PipelineRegister62/1 -> _adder_MultiplyAdd_out_dtc62/1
  PipelineRegister61/1 -> _adder_MultiplyAdd_out_dtc61/1
  PipelineRegister60/1 -> _adder_MultiplyAdd_out_dtc60/1
  PipelineRegister59/1 -> _adder_MultiplyAdd_out_dtc59/1
  PipelineRegister58/1 -> _adder_MultiplyAdd_out_dtc58/1
  PipelineRegister57/1 -> _adder_MultiplyAdd_out_dtc57/1
  PipelineRegister56/1 -> _adder_MultiplyAdd_out_dtc56/1
  PipelineRegister55/1 -> _adder_MultiplyAdd_out_dtc55/1
  PipelineRegister54/1 -> _adder_MultiplyAdd_out_dtc54/1
  PipelineRegister53/1 -> _adder_MultiplyAdd_out_dtc53/1
  PipelineRegister52/1 -> _adder_MultiplyAdd_out_dtc52/1
  PipelineRegister51/1 -> _adder_MultiplyAdd_out_dtc51/1
  PipelineRegister50/1 -> _adder_MultiplyAdd_out_dtc50/1
  PipelineRegister49/1 -> _adder_MultiplyAdd_out_dtc49/1
  PipelineRegister48/1 -> _adder_MultiplyAdd_out_dtc48/1
  PipelineRegister47/1 -> _adder_MultiplyAdd_out_dtc47/1
  PipelineRegister46/1 -> _adder_MultiplyAdd_out_dtc46/1
  PipelineRegister45/1 -> _adder_MultiplyAdd_out_dtc45/1
  PipelineRegister44/1 -> _adder_MultiplyAdd_out_dtc44/1
  PipelineRegister43/1 -> _adder_MultiplyAdd_out_dtc43/1
  PipelineRegister42/1 -> _adder_MultiplyAdd_out_dtc42/1
  PipelineRegister41/1 -> _adder_MultiplyAdd_out_dtc41/1
  PipelineRegister40/1 -> _adder_MultiplyAdd_out_dtc40/1
  PipelineRegister39/1 -> _adder_MultiplyAdd_out_dtc39/1
  PipelineRegister38/1 -> _adder_MultiplyAdd_out_dtc38/1
  PipelineRegister37/1 -> _adder_MultiplyAdd_out_dtc37/1
  PipelineRegister36/1 -> _adder_MultiplyAdd_out_dtc36/1
  PipelineRegister35/1 -> _adder_MultiplyAdd_out_dtc35/1
  PipelineRegister34/1 -> _adder_MultiplyAdd_out_dtc34/1
  PipelineRegister33/1 -> _adder_MultiplyAdd_out_dtc33/1
  PipelineRegister32/1 -> _adder_MultiplyAdd_out_dtc32/1
  PipelineRegister31/1 -> _adder_MultiplyAdd_out_dtc31/1
  PipelineRegister30/1 -> _adder_MultiplyAdd_out_dtc30/1
  PipelineRegister29/1 -> _adder_MultiplyAdd_out_dtc29/1
  PipelineRegister28/1 -> _adder_MultiplyAdd_out_dtc28/1
  PipelineRegister27/1 -> _adder_MultiplyAdd_out_dtc27/1
  PipelineRegister26/1 -> _adder_MultiplyAdd_out_dtc26/1
  PipelineRegister25/1 -> _adder_MultiplyAdd_out_dtc25/1
  PipelineRegister24/1 -> _adder_MultiplyAdd_out_dtc24/1
  PipelineRegister23/1 -> _adder_MultiplyAdd_out_dtc23/1
  PipelineRegister22/1 -> _adder_MultiplyAdd_out_dtc22/1
  PipelineRegister21/1 -> _adder_MultiplyAdd_out_dtc21/1
  PipelineRegister20/1 -> _adder_MultiplyAdd_out_dtc20/1
  PipelineRegister19/1 -> _adder_MultiplyAdd_out_dtc19/1
  PipelineRegister18/1 -> _adder_MultiplyAdd_out_dtc18/1
  PipelineRegister17/1 -> _adder_MultiplyAdd_out_dtc17/1
  PipelineRegister16/1 -> _adder_MultiplyAdd_out_dtc16/1
  PipelineRegister15/1 -> _adder_MultiplyAdd_out_dtc15/1
  PipelineRegister14/1 -> _adder_MultiplyAdd_out_dtc14/1
  PipelineRegister13/1 -> _adder_MultiplyAdd_out_dtc13/1
  PipelineRegister12/1 -> _adder_MultiplyAdd_out_dtc12/1
  PipelineRegister11/1 -> _adder_MultiplyAdd_out_dtc11/1
  PipelineRegister10/1 -> _adder_MultiplyAdd_out_dtc10/1
  PipelineRegister9/1 -> _adder_MultiplyAdd_out_dtc9/1
  PipelineRegister8/1 -> _adder_MultiplyAdd_out_dtc8/1
  PipelineRegister7/1 -> _adder_MultiplyAdd_out_dtc7/1
  PipelineRegister6/1 -> _adder_MultiplyAdd_out_dtc6/1
  PipelineRegister5/1 -> _adder_MultiplyAdd_out_dtc5/1
  PipelineRegister4/1 -> _adder_MultiplyAdd_out_dtc4/1
  PipelineRegister3/1 -> _adder_MultiplyAdd_out_dtc3/1
  PipelineRegister2/1 -> _adder_MultiplyAdd_out_dtc2/1
  PipelineRegister1/1 -> _adder_MultiplyAdd_out_dtc1/1
  PipelineRegister/1 -> _adder_MultiplyAdd_out_dtc/1
  _adder_MultiplyAdd_out_dtc79/1 -> HwModeRegister242/1
  delayMatch143/1 -> HwModeRegister241/1
  delayMatch142/1 -> HwModeRegister240/1
  _adder_MultiplyAdd_out_dtc78/1 -> HwModeRegister239/1
  delayMatch125/1 -> HwModeRegister238/1
  delayMatch124/1 -> HwModeRegister237/1
  _adder_MultiplyAdd_out_dtc77/1 -> HwModeRegister236/1
  delayMatch123/1 -> HwModeRegister235/1
  delayMatch122/1 -> HwModeRegister234/1
  _adder_MultiplyAdd_out_dtc76/1 -> HwModeRegister233/1
  delayMatch121/1 -> HwModeRegister232/1
  delayMatch120/1 -> HwModeRegister231/1
  _adder_MultiplyAdd_out_dtc75/1 -> HwModeRegister230/1
  delayMatch119/1 -> HwModeRegister229/1
  delayMatch118/1 -> HwModeRegister228/1
  _adder_MultiplyAdd_out_dtc74/1 -> HwModeRegister227/1
  delayMatch117/1 -> HwModeRegister226/1
  delayMatch116/1 -> HwModeRegister225/1
  _adder_MultiplyAdd_out_dtc73/1 -> HwModeRegister224/1
  delayMatch115/1 -> HwModeRegister223/1
  delayMatch114/1 -> HwModeRegister222/1
  _adder_MultiplyAdd_out_dtc72/1 -> HwModeRegister221/1
  delayMatch113/1 -> HwModeRegister220/1
  delayMatch112/1 -> HwModeRegister219/1
  t23/1 -> HwModeRegister217/1
  t22/1 -> HwModeRegister216/1
  _bias8/1 -> HwModeRegister218/1
  _adder_MultiplyAdd_out_dtc70/1 -> HwModeRegister215/1
  delayMatch141/1 -> HwModeRegister214/1
  delayMatch140/1 -> HwModeRegister213/1
  _adder_MultiplyAdd_out_dtc69/1 -> HwModeRegister212/1
  delayMatch111/1 -> HwModeRegister211/1
  delayMatch110/1 -> HwModeRegister210/1
  _adder_MultiplyAdd_out_dtc68/1 -> HwModeRegister209/1
  delayMatch109/1 -> HwModeRegister208/1
  delayMatch108/1 -> HwModeRegister207/1
  _adder_MultiplyAdd_out_dtc67/1 -> HwModeRegister206/1
  delayMatch107/1 -> HwModeRegister205/1
  delayMatch106/1 -> HwModeRegister204/1
  _adder_MultiplyAdd_out_dtc66/1 -> HwModeRegister203/1
  delayMatch105/1 -> HwModeRegister202/1
  delayMatch104/1 -> HwModeRegister201/1
  _adder_MultiplyAdd_out_dtc65/1 -> HwModeRegister200/1
  delayMatch103/1 -> HwModeRegister199/1
  delayMatch102/1 -> HwModeRegister198/1
  _adder_MultiplyAdd_out_dtc64/1 -> HwModeRegister197/1
  delayMatch101/1 -> HwModeRegister196/1
  delayMatch100/1 -> HwModeRegister195/1
  _adder_MultiplyAdd_out_dtc63/1 -> HwModeRegister194/1
  delayMatch99/1 -> HwModeRegister193/1
  delayMatch98/1 -> HwModeRegister192/1
  t21/1 -> HwModeRegister190/1
  t20/1 -> HwModeRegister189/1
  _bias7/1 -> HwModeRegister191/1
  _adder_MultiplyAdd_out_dtc61/1 -> HwModeRegister188/1
  delayMatch139/1 -> HwModeRegister187/1
  delayMatch138/1 -> HwModeRegister186/1
  _adder_MultiplyAdd_out_dtc60/1 -> HwModeRegister185/1
  delayMatch97/1 -> HwModeRegister184/1
  delayMatch96/1 -> HwModeRegister183/1
  _adder_MultiplyAdd_out_dtc59/1 -> HwModeRegister182/1
  delayMatch95/1 -> HwModeRegister181/1
  delayMatch94/1 -> HwModeRegister180/1
  _adder_MultiplyAdd_out_dtc58/1 -> HwModeRegister179/1
  delayMatch93/1 -> HwModeRegister178/1
  delayMatch92/1 -> HwModeRegister177/1
  _adder_MultiplyAdd_out_dtc57/1 -> HwModeRegister176/1
  delayMatch91/1 -> HwModeRegister175/1
  delayMatch90/1 -> HwModeRegister174/1
  _adder_MultiplyAdd_out_dtc56/1 -> HwModeRegister173/1
  delayMatch89/1 -> HwModeRegister172/1
  delayMatch88/1 -> HwModeRegister171/1
  _adder_MultiplyAdd_out_dtc55/1 -> HwModeRegister170/1
  delayMatch87/1 -> HwModeRegister169/1
  delayMatch86/1 -> HwModeRegister168/1
  _adder_MultiplyAdd_out_dtc54/1 -> HwModeRegister167/1
  delayMatch85/1 -> HwModeRegister166/1
  delayMatch84/1 -> HwModeRegister165/1
  t19/1 -> HwModeRegister163/1
  t18/1 -> HwModeRegister162/1
  _bias6/1 -> HwModeRegister164/1
  _adder_MultiplyAdd_out_dtc52/1 -> HwModeRegister161/1
  delayMatch137/1 -> HwModeRegister160/1
  delayMatch136/1 -> HwModeRegister159/1
  _adder_MultiplyAdd_out_dtc51/1 -> HwModeRegister158/1
  delayMatch83/1 -> HwModeRegister157/1
  delayMatch82/1 -> HwModeRegister156/1
  _adder_MultiplyAdd_out_dtc50/1 -> HwModeRegister155/1
  delayMatch81/1 -> HwModeRegister154/1
  delayMatch80/1 -> HwModeRegister153/1
  _adder_MultiplyAdd_out_dtc49/1 -> HwModeRegister152/1
  delayMatch79/1 -> HwModeRegister151/1
  delayMatch78/1 -> HwModeRegister150/1
  _adder_MultiplyAdd_out_dtc48/1 -> HwModeRegister149/1
  delayMatch77/1 -> HwModeRegister148/1
  delayMatch76/1 -> HwModeRegister147/1
  _adder_MultiplyAdd_out_dtc47/1 -> HwModeRegister146/1
  delayMatch75/1 -> HwModeRegister145/1
  delayMatch74/1 -> HwModeRegister144/1
  _adder_MultiplyAdd_out_dtc46/1 -> HwModeRegister143/1
  delayMatch73/1 -> HwModeRegister142/1
  delayMatch72/1 -> HwModeRegister141/1
  _adder_MultiplyAdd_out_dtc45/1 -> HwModeRegister140/1
  delayMatch71/1 -> HwModeRegister139/1
  delayMatch70/1 -> HwModeRegister138/1
  t17/1 -> HwModeRegister136/1
  t16/1 -> HwModeRegister135/1
  _bias5/1 -> HwModeRegister137/1
  _adder_MultiplyAdd_out_dtc43/1 -> HwModeRegister134/1
  delayMatch135/1 -> HwModeRegister133/1
  delayMatch134/1 -> HwModeRegister132/1
  _adder_MultiplyAdd_out_dtc42/1 -> HwModeRegister131/1
  delayMatch69/1 -> HwModeRegister130/1
  delayMatch68/1 -> HwModeRegister129/1
  _adder_MultiplyAdd_out_dtc41/1 -> HwModeRegister128/1
  delayMatch67/1 -> HwModeRegister127/1
  delayMatch66/1 -> HwModeRegister126/1
  _adder_MultiplyAdd_out_dtc40/1 -> HwModeRegister125/1
  delayMatch65/1 -> HwModeRegister124/1
  delayMatch64/1 -> HwModeRegister123/1
  _adder_MultiplyAdd_out_dtc39/1 -> HwModeRegister122/1
  delayMatch63/1 -> HwModeRegister121/1
  delayMatch62/1 -> HwModeRegister120/1
  _adder_MultiplyAdd_out_dtc38/1 -> HwModeRegister119/1
  delayMatch61/1 -> HwModeRegister118/1
  delayMatch60/1 -> HwModeRegister117/1
  _adder_MultiplyAdd_out_dtc37/1 -> HwModeRegister116/1
  delayMatch59/1 -> HwModeRegister115/1
  delayMatch58/1 -> HwModeRegister114/1
  _adder_MultiplyAdd_out_dtc36/1 -> HwModeRegister113/1
  delayMatch57/1 -> HwModeRegister112/1
  delayMatch56/1 -> HwModeRegister111/1
  t15/1 -> HwModeRegister109/1
  t14/1 -> HwModeRegister108/1
  _bias4/1 -> HwModeRegister110/1
  _adder_MultiplyAdd_out_dtc34/1 -> HwModeRegister107/1
  delayMatch133/1 -> HwModeRegister106/1
  delayMatch132/1 -> HwModeRegister105/1
  _adder_MultiplyAdd_out_dtc33/1 -> HwModeRegister104/1
  delayMatch55/1 -> HwModeRegister103/1
  delayMatch54/1 -> HwModeRegister102/1
  _adder_MultiplyAdd_out_dtc32/1 -> HwModeRegister101/1
  delayMatch53/1 -> HwModeRegister100/1
  delayMatch52/1 -> HwModeRegister99/1
  _adder_MultiplyAdd_out_dtc31/1 -> HwModeRegister98/1
  delayMatch51/1 -> HwModeRegister97/1
  delayMatch50/1 -> HwModeRegister96/1
  _adder_MultiplyAdd_out_dtc30/1 -> HwModeRegister95/1
  delayMatch49/1 -> HwModeRegister94/1
  delayMatch48/1 -> HwModeRegister93/1
  _adder_MultiplyAdd_out_dtc29/1 -> HwModeRegister92/1
  delayMatch47/1 -> HwModeRegister91/1
  delayMatch46/1 -> HwModeRegister90/1
  _adder_MultiplyAdd_out_dtc28/1 -> HwModeRegister89/1
  delayMatch45/1 -> HwModeRegister88/1
  delayMatch44/1 -> HwModeRegister87/1
  _adder_MultiplyAdd_out_dtc27/1 -> HwModeRegister86/1
  delayMatch43/1 -> HwModeRegister85/1
  delayMatch42/1 -> HwModeRegister84/1
  t13/1 -> HwModeRegister82/1
  t12/1 -> HwModeRegister81/1
  _bias3/1 -> HwModeRegister83/1
  _adder_MultiplyAdd_out_dtc25/1 -> HwModeRegister80/1
  delayMatch131/1 -> HwModeRegister79/1
  delayMatch130/1 -> HwModeRegister78/1
  _adder_MultiplyAdd_out_dtc24/1 -> HwModeRegister77/1
  delayMatch41/1 -> HwModeRegister76/1
  delayMatch40/1 -> HwModeRegister75/1
  _adder_MultiplyAdd_out_dtc23/1 -> HwModeRegister74/1
  delayMatch39/1 -> HwModeRegister73/1
  delayMatch38/1 -> HwModeRegister72/1
  _adder_MultiplyAdd_out_dtc22/1 -> HwModeRegister71/1
  delayMatch37/1 -> HwModeRegister70/1
  delayMatch36/1 -> HwModeRegister69/1
  _adder_MultiplyAdd_out_dtc21/1 -> HwModeRegister68/1
  delayMatch35/1 -> HwModeRegister67/1
  delayMatch34/1 -> HwModeRegister66/1
  _adder_MultiplyAdd_out_dtc20/1 -> HwModeRegister65/1
  delayMatch33/1 -> HwModeRegister64/1
  delayMatch32/1 -> HwModeRegister63/1
  _adder_MultiplyAdd_out_dtc19/1 -> HwModeRegister62/1
  delayMatch31/1 -> HwModeRegister61/1
  delayMatch30/1 -> HwModeRegister60/1
  _adder_MultiplyAdd_out_dtc18/1 -> HwModeRegister59/1
  delayMatch29/1 -> HwModeRegister58/1
  delayMatch28/1 -> HwModeRegister57/1
  t11/1 -> HwModeRegister55/1
  t10/1 -> HwModeRegister54/1
  _bias2/1 -> HwModeRegister56/1
  _adder_MultiplyAdd_out_dtc16/1 -> HwModeRegister53/1
  delayMatch129/1 -> HwModeRegister52/1
  delayMatch128/1 -> HwModeRegister51/1
  _adder_MultiplyAdd_out_dtc15/1 -> HwModeRegister50/1
  delayMatch27/1 -> HwModeRegister49/1
  delayMatch26/1 -> HwModeRegister48/1
  _adder_MultiplyAdd_out_dtc14/1 -> HwModeRegister47/1
  delayMatch25/1 -> HwModeRegister46/1
  delayMatch24/1 -> HwModeRegister45/1
  _adder_MultiplyAdd_out_dtc13/1 -> HwModeRegister44/1
  delayMatch23/1 -> HwModeRegister43/1
  delayMatch22/1 -> HwModeRegister42/1
  _adder_MultiplyAdd_out_dtc12/1 -> HwModeRegister41/1
  delayMatch21/1 -> HwModeRegister40/1
  delayMatch20/1 -> HwModeRegister39/1
  _adder_MultiplyAdd_out_dtc11/1 -> HwModeRegister38/1
  delayMatch19/1 -> HwModeRegister37/1
  delayMatch18/1 -> HwModeRegister36/1
  _adder_MultiplyAdd_out_dtc10/1 -> HwModeRegister35/1
  delayMatch17/1 -> HwModeRegister34/1
  delayMatch16/1 -> HwModeRegister33/1
  _adder_MultiplyAdd_out_dtc9/1 -> HwModeRegister32/1
  delayMatch15/1 -> HwModeRegister31/1
  delayMatch14/1 -> HwModeRegister30/1
  t9/1 -> HwModeRegister28/1
  t8/1 -> HwModeRegister27/1
  _bias1/1 -> HwModeRegister29/1
  _adder_MultiplyAdd_out_dtc7/1 -> HwModeRegister26/1
  delayMatch127/1 -> HwModeRegister25/1
  delayMatch126/1 -> HwModeRegister24/1
  _adder_MultiplyAdd_out_dtc6/1 -> HwModeRegister23/1
  delayMatch13/1 -> HwModeRegister22/1
  delayMatch12/1 -> HwModeRegister21/1
  _adder_MultiplyAdd_out_dtc5/1 -> HwModeRegister20/1
  delayMatch11/1 -> HwModeRegister19/1
  delayMatch10/1 -> HwModeRegister18/1
  _adder_MultiplyAdd_out_dtc4/1 -> HwModeRegister17/1
  delayMatch9/1 -> HwModeRegister16/1
  delayMatch8/1 -> HwModeRegister15/1
  _adder_MultiplyAdd_out_dtc3/1 -> HwModeRegister14/1
  delayMatch7/1 -> HwModeRegister13/1
  delayMatch6/1 -> HwModeRegister12/1
  _adder_MultiplyAdd_out_dtc2/1 -> HwModeRegister11/1
  delayMatch5/1 -> HwModeRegister10/1
  delayMatch4/1 -> HwModeRegister9/1
  _adder_MultiplyAdd_out_dtc1/1 -> HwModeRegister8/1
  delayMatch3/1 -> HwModeRegister7/1
  delayMatch2/1 -> HwModeRegister6/1
  _adder_MultiplyAdd_out_dtc/1 -> HwModeRegister5/1
  delayMatch1/1 -> HwModeRegister4/1
  delayMatch/1 -> HwModeRegister3/1
  t7/1 -> HwModeRegister1/1
  t6/1 -> HwModeRegister/1
  _bias/1 -> HwModeRegister2/1
  t4/1 -> t5/1
  _adder_MultiplyAdd_out_dtc80/1 -> t4/9
  _adder_MultiplyAdd_out_dtc71/1 -> t4/8
  _adder_MultiplyAdd_out_dtc62/1 -> t4/7
  _adder_MultiplyAdd_out_dtc53/1 -> t4/6
  _adder_MultiplyAdd_out_dtc44/1 -> t4/5
  _adder_MultiplyAdd_out_dtc35/1 -> t4/4
  _adder_MultiplyAdd_out_dtc26/1 -> t4/3
  _adder_MultiplyAdd_out_dtc17/1 -> t4/2
  _adder_MultiplyAdd_out_dtc8/1 -> t4/1
  t3/9(out8) -> t22/1
  t3/8(out7) -> t20/1
  t3/7(out6) -> t18/1
  t3/6(out5) -> t16/1
  t3/5(out4) -> t14/1
  t3/4(out3) -> t12/1
  t3/3(out2) -> t10/1
  t3/2(out1) -> t8/1
  t3/1(out0) -> t6/1
  t2/1 -> t3/1(in0)
  Constant1/1 -> t1/1
  t/9 -> delayMatch158/1
  t/8 -> delayMatch157/1
  t/7 -> delayMatch156/1
  t/6 -> delayMatch155/1
  t/5 -> delayMatch154/1
  t/4 -> delayMatch153/1
  t/3 -> delayMatch152/1
  t/2 -> Data Type Conversion39_out1_1_wire/1
  t/1 -> Data Type Conversion39_out1_0_wire/1
  mux/1 -> out/1
  t5/1 -> Data Type Conversion39/1(In1)
  delayMatch150/1 -> Divide3/1(In1)
  delayMatch149/1 -> Divide1/1(In1)
  delayMatch148/1 -> Divide/1(In1)
  delayMatch151/1 -> Divide2/1(In1)
  delayMatch158/1 -> mux/9
  delayMatch157/1 -> mux/8
  delayMatch156/1 -> mux/7
  delayMatch155/1 -> mux/6
  delayMatch154/1 -> mux/5
  delayMatch153/1 -> mux/4
  delayMatch152/1 -> mux/3
  Data Type Conversion39_out1_1_wire/1 -> Divide1/2(In2), Divide3/2(In2)
  Data Type Conversion39_out1_0_wire/1 -> Divide/2(In2), Divide2/2(In2)
  t1/1 -> t2/1

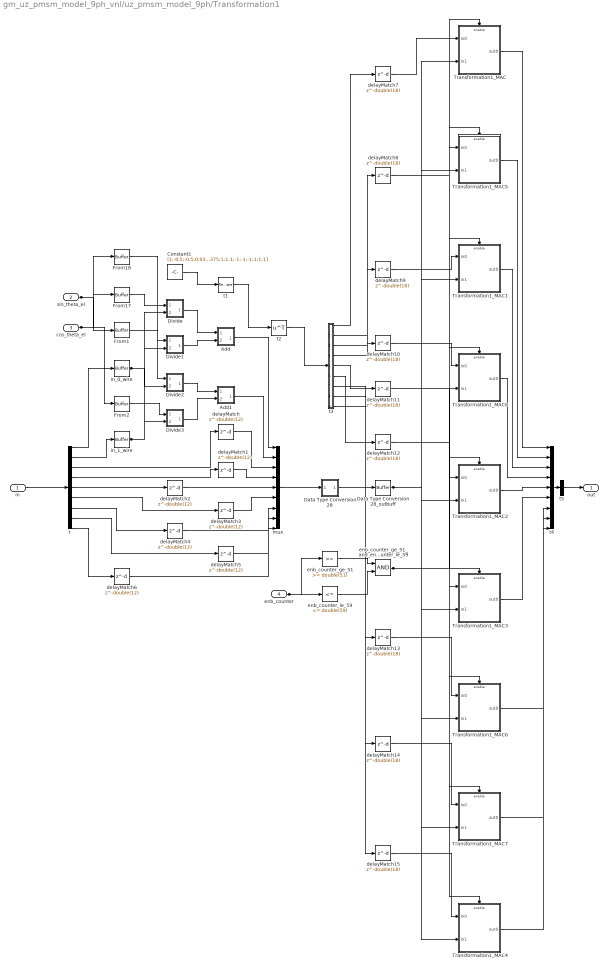
== system gm_uz_pmsm_model_9ph_vnl/uz_pmsm_model_9ph/Transformation1 ==
  in : Inport  OutDataTypeStr=single  PortDimensions=[9]  SampleTime=1e-08
  sin_theta_el : Inport  Port=2  OutDataTypeStr=single  SampleTime=1e-08
  cos_theta_el : Inport  Port=3  OutDataTypeStr=single  SampleTime=1e-08
  enb_counter : Inport  Port=4  OutDataTypeStr=uint8  SampleTime=1e-08
  Add : Subsystem
      mask Display: disp('NFP\nadd');
  Add1 : Subsystem
      mask Display: disp('NFP\nadd');
  Constant1 : Constant  Value=[1;-0.5;-0.5;0.939697265625;-0.7660369873046875;-0.17364501953125;0.7660369873046875;-0.939697265625;0.17364501953125;0;0.86602783203125;-0.86602783203125;0.3420257568359375;0.642791748046875;-0.98480224609375;0.642791748046875;0.3420257568359375;-0.98480224609375;1;1;1;0.5;0.5;0.5;-0.5;-0.5;-0.5;0;0;0;0.86602783203125;0.86602783203125;0.86602783203125;0.86602783203125;0.86602783203125;0.86602783203125;1;-0.5;-0.5;-0.17364501953125;0.939697265625;-0.7660369873046875;-0.939697265625;0.17364501953125;0.7660369873046875;0;-0.86602783203125;0.86602783203125;0.98480224609375;-0.3420257568359375;-0.642791748046875;-0.3420257568359375;0.98480224609375;-0.642791748046875;1;-0.5;-0.5;-0.7660369873046875;-0.17364501953125;0.939697265625;0.17364501953125;0.7660369873046875;-0.939697265625;0;0.86602783203125;-0.86602783203125;0.642791748046875;-0.98480224609375;0.3420257568359375;-0.98480224609375;0.642791748046875;0.3420257568359375;1;1;1;-1;-1;-1;1;1;1]  OutDataTypeStr=fixdt(1, 18, 16)  SampleTime=1e-08
  Data Type Conversion28 : Subsystem
      mask Display: disp('NFP\nconv');
  Data Type Conversion28_outbuff : hdlmdlgenlib/Buffer
      settings: SourceProductBaseCode=SL
  Divide : Subsystem
      mask Display: disp('NFP\nmul');
  Divide1 : Subsystem
      mask Display: disp('NFP\nmul');
  Divide2 : Subsystem
      mask Display: disp('NFP\nmul');
  Divide3 : Subsystem
      mask Display: disp('NFP\nmul');
  From{1..2,17..18} (4 alike) : hdlmdlgenlib/Buffer
      settings: SourceProductBaseCode=SL
  Transformation1_MAC : Subsystem
      settings: MinAlgLoopOccurrences=on
  Transformation1_MAC1 : Subsystem
      settings: MinAlgLoopOccurrences=on
  Transformation1_MAC2 : Subsystem
      settings: MinAlgLoopOccurrences=on
  Transformation1_MAC3 : Subsystem
      settings: MinAlgLoopOccurrences=on
  Transformation1_MAC4 : Subsystem
      settings: MinAlgLoopOccurrences=on
  Transformation1_MAC5 : Subsystem
      settings: MinAlgLoopOccurrences=on
  Transformation1_MAC6 : Subsystem
      settings: MinAlgLoopOccurrences=on
  Transformation1_MAC7 : Subsystem
      settings: MinAlgLoopOccurrences=on
  Transformation1_MAC8 : Subsystem
      settings: MinAlgLoopOccurrences=on
  delayMatch{,1..6} (7 alike) : Delay  DelayLength=double(12)  InitialCondition=0  SampleTime=1e-08
  delayMatch{7..15} (9 alike) : Delay  DelayLength=double(18)  InitialCondition=0  SampleTime=1e-08
  enb_counter_ge_51 : simulink/Logic and Bit Operations/Compare To Constant  relop=>=  const=double(51)  OutDataTypeStr=boolean
  enb_counter_ge_51_and_enb_counter_le_59 : Logic  AllPortsSameDT=off  OutDataTypeStr=boolean  SampleTime=1e-08
  enb_counter_le_59 : simulink/Logic and Bit Operations/Compare To Constant  relop=<=  const=double(59)  OutDataTypeStr=boolean
  in_0_wire : hdlmdlgenlib/Buffer
      settings: SourceProductBaseCode=SL
  in_1_wire : hdlmdlgenlib/Buffer
      settings: SourceProductBaseCode=SL
  mux : Mux  Inputs=9
  t : Demux  Outputs=9
  t1 : Reshape  OutputDimensionality=Customize  OutputDimensions=[9,9]
  t2 : Math  Operator=transpose  SaturateOnIntegerOverflow=on
  t3 : Subsystem
  t4 : Mux  Inputs=9
  t5 : Concatenate  NumInputs=1  Mode=Multidimensional array  ConcatenateDimension=2
  out : Outport  SampleTime=1e-08
  wires:
  enb_counter/1 -> enb_counter_ge_51/1, enb_counter_le_59/1
  cos_theta_el/1 -> From17/1, From2/1
  sin_theta_el/1 -> From1/1, From18/1
  in/1 -> t/1
  enb_counter_le_59/1 -> enb_counter_ge_51_and_enb_counter_le_59/2
  enb_counter_ge_51/1 -> enb_counter_ge_51_and_enb_counter_le_59/1
  enb_counter_ge_51_and_enb_counter_le_59/1 -> Transformation1_MAC/Enable, Transformation1_MAC1/Enable, Transformation1_MAC2/Enable, Transformation1_MAC3/Enable, Transformation1_MAC4/Enable, Transformation1_MAC5/Enable, Transformation1_MAC6/Enable, Transformation1_MAC7/Enable, Transformation1_MAC8/Enable
  t3/9(out8) -> delayMatch15/1
  t3/8(out7) -> delayMatch14/1
  t3/7(out6) -> delayMatch13/1
  t3/6(out5) -> delayMatch12/1
  t3/5(out4) -> delayMatch11/1
  t3/4(out3) -> delayMatch10/1
  t3/3(out2) -> delayMatch9/1
  t3/2(out1) -> delayMatch8/1
  t3/1(out0) -> delayMatch7/1
  Divide3/1(Out1) -> Add1/2(In2)
  Divide2/1(Out1) -> Add1/1(In1)
  Divide1/1(Out1) -> Add/2(In2)
  Divide/1(Out1) -> Add/1(In1)
  Data Type Conversion28/1(Out1) -> Data Type Conversion28_outbuff/1
  Add1/1(Out1) -> mux/2
  Add/1(Out1) -> mux/1
  t4/1 -> t5/1
  Transformation1_MAC4/1(out0) -> t4/9
  Transformation1_MAC7/1(out0) -> t4/8
  Transformation1_MAC6/1(out0) -> t4/7
  Transformation1_MAC3/1(out0) -> t4/6
  Transformation1_MAC2/1(out0) -> t4/5
  Transformation1_MAC8/1(out0) -> t4/4
  Transformation1_MAC1/1(out0) -> t4/3
  Transformation1_MAC5/1(out0) -> t4/2
  Transformation1_MAC/1(out0) -> t4/1
  delayMatch15/1 -> Transformation1_MAC4/1(in0)
  delayMatch14/1 -> Transformation1_MAC7/1(in0)
  delayMatch13/1 -> Transformation1_MAC6/1(in0)
  delayMatch12/1 -> Transformation1_MAC3/1(in0)
  delayMatch11/1 -> Transformation1_MAC2/1(in0)
  delayMatch10/1 -> Transformation1_MAC8/1(in0)
  delayMatch9/1 -> Transformation1_MAC1/1(in0)
  delayMatch8/1 -> Transformation1_MAC5/1(in0)
  delayMatch7/1 -> Transformation1_MAC/1(in0)
  t2/1 -> t3/1(in0)
  Constant1/1 -> t1/1
  t/9 -> delayMatch6/1
  t/8 -> delayMatch5/1
  t/7 -> delayMatch4/1
  t/6 -> delayMatch3/1
  t/5 -> delayMatch2/1
  t/4 -> delayMatch1/1
  t/3 -> delayMatch/1
  t/2 -> in_1_wire/1
  t/1 -> in_0_wire/1
  mux/1 -> Data Type Conversion28/1(In1)
  t5/1 -> out/1
  From2/1 -> Divide3/1(In1)
  From18/1 -> Divide1/1(In1)
  From17/1 -> Divide/1(In1)
  From1/1 -> Divide2/1(In1)
  delayMatch6/1 -> mux/9
  delayMatch5/1 -> mux/8
  delayMatch4/1 -> mux/7
  delayMatch3/1 -> mux/6
  delayMatch2/1 -> mux/5
  delayMatch1/1 -> mux/4
  delayMatch/1 -> mux/3
  in_1_wire/1 -> Divide1/2(In2), Divide3/2(In2)
  in_0_wire/1 -> Divide/2(In2), Divide2/2(In2)
  Data Type Conversion28_outbuff/1 -> Transformation1_MAC/2(in1), Transformation1_MAC1/2(in1), Transformation1_MAC2/2(in1), Transformation1_MAC3/2(in1), Transformation1_MAC4/2(in1), Transformation1_MAC5/2(in1), Transformation1_MAC6/2(in1), Transformation1_MAC7/2(in1), Transformation1_MAC8/2(in1)
  t1/1 -> t2/1
